simulink model "househeat"  (R2018b)
settings: Solver=ode15s  StartTime=0.0  StopTime=3600*24*55  FixedStep=1  RelTol=1e-3  AbsTol=1e-6
model workspace (MATLAB code in the model file):
  | % load initial conditions and physical properties from file
  | 
  | %sldemo_househeat_data
  | househeat_data_szakdoga
  | onlabmpc
  | 
  | 
  | addpath('subsystems')
  | 
  | %disp('adding models...')
  | load('subsystems/MPC-expert.mat')
  | %disp('done.')
values from neighbouring files (symbols this model uses):
  A_heater = 3.5    [househeat_data_szakdoga.m]
  c = 1005.4    [househeat_data_szakdoga.m]
  h_heater = 11    [househeat_data_szakdoga.m]
  M = (lenHouse*widHouse*htHouse+tan(pitRoof)*widHouse*lenHouse)*densAir    [househeat_data_szakdoga.m]
  Req = RWall*RWindow/(RWall + RWindow)    [househeat_data_szakdoga.m]
  T_s = 1800    [househeat_data_szakdoga.m]
  timeUnit_1week = 7*timeUnit_1day    (= 336)    [househeat_data_szakdoga.m]
  TinHeatK = 273    [househeat_data_szakdoga.m]
  TinIC = 0    [househeat_data_szakdoga.m]
undefined symbols (not defined in the file or in its folder): disturbance, f, FloorHeatFlowIn, RadiatorHeatFlow, RadiatorSurface, referenceSloped
libraries: fl_lib x39, nesl_utility x14, simulink x2, instrumentlib x2, mpclib x1, dspnetwork x1, powerlib_meascontrol x1
Description:
  | Thermal Model of a House
  | 
  | This demo illustrates how you can use Simulink(R) to create the thermal model of
  | a house. This system models the outdoor environment, the thermal
  | characteristics of the house, and the house heating system.
  | 
  | The sldemo_househeat_data.m file initializes data in the model workspace.
  | To make changes, you can edit the model workspace directly or edit the MATLAB(R) file
  | and re-load the model workspace.
  | 
  | To view the model workspace, select View > Model Explorer
  | from the Simulink editor.
  | 
  | Note: Time is given in units of hours
settings Model: SimulationMode=accelerator  PauseTimes=648000  NumberOfSteps=100  ExtModeTrigMode=oneshot  ExtModeArmWhenConnect=off  ExtModeAutoUpdateStatusClock=off  Creator=The MathWorks, Inc.  LastModifiedBy=Gyulai László
settings SolverCC: AutoScaleAbsTol=off
settings DataIOCC: ExternalInput=[]  InitialState=[]  SaveFormat=StructureWithTime  SaveOutput=off  SaveTime=off  SignalLoggingName=sldemo_househeat_output
settings OptimizationCC: BlockReduction=off  BooleanDataType=off  ExpressionDepthLimit=2147483647  InitFltsAndDblsToZero=on  EfficientMapNaN2IntZero=off  LifeSpan=inf  BufferReusableBoundary=off
settings DebuggingCC: SaveWithParameterizedLinksMsg=none  UnderspecifiedInitializationDetection=Classic  MergeDetectMultiDrivingBlocksExec=none  SignalResolutionControl=TryResolveAllWithWarning  MultiTaskDSMMsg=warning  MultiTaskCondExecSysMsg=none  IntegerOverflowMsg=none  FcnCallInpInsideContextMsg=warning  BusObjectLabelMismatch=none  StateNameClashWarn=warning  SFUnexpectedBacktrackingDiag=warning  SFNoUnconditionalDefaultTransitionDiag=warning  SFExecutionAtInitializationDiag=none  IntegerSaturationMsg=none
settings HardwareCC: ProdBitPerPointer=32  ProdBitPerSizeT=32  ProdBitPerPtrDiffT=32  ProdLargestAtomicFloat=None  ProdIntDivRoundTo=Undefined  ProdEndianess=Unspecified  ProdWordSize=32  ProdHWDeviceType=32-bit Generic  TargetBitPerPointer=64  TargetBitPerSizeT=64  TargetBitPerPtrDiffT=64  TargetLongLongMode=on  TargetIntDivRoundTo=Zero  TargetEndianess=LittleEndian  TargetWordSize=64  TargetHWDeviceType=MATLAB Host  ProdEqTarget=off
settings ModelReferenceCC: PropagateSignalLabelsOutOfModel=off
settings SFSimCC: SimUseLocalCustomCode=off
settings CodeAppCC: MaxIdLength=128
settings GRTTargetCC: TargetLangStandard=C89/C90 (ANSI)  CombineOutputUpdateFcns=off  GRTInterface=on
settings ConfigComp: CovMetricSettings=dw  CovHtmlReporting=on  CovSaveCumulativeToWorkspaceVar=on  CovSaveSingleToWorkspaceVar=on  CovExternalEMLEnable=off
settings SimscapeCC: SimscapeNormalizeSystem=off

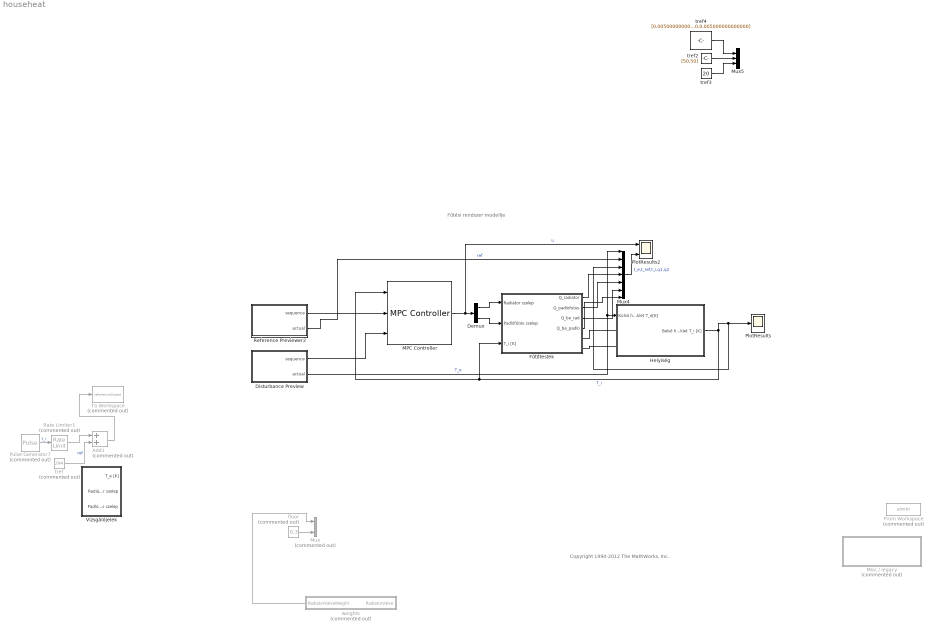
== system househeat ==
  note: Fűtési rendszer modellje
  note: Copyright 1990-2012 The MathWorks, Inc.
  Add1 : Sum  Commented=on
  Demux : Demux  Outputs=2
  Disturbance Preview : Subsystem  mask{signal=disturbance, ts=1800, steps=10}
      mask prompts: signal "Signal name"; ts "Sampling time"; steps "Number of previewing steps"
      mask init:
      | ts = evalin('base',get_param(gcbh,'ts'));
      | signal = evalin('base',get_param(gcbh,'signal'));
      | steps = evalin('base',get_param(gcbh,'steps'));
      | data = mpc_previewer_maskinit(signal,ts);
      mask Display:
      | fprintf('Future\nsample\nextractor');
      | port_label('output', 1, 'seq')
      | port_label('output', 2, '@t')
  From Workspace : FromWorkspace  Commented=on  VariableName=simin  SampleTime=0
  Fűtőtestek : Subsystem
  Helyiség : Subsystem
  MPC Controller : mpclib/MPC Controller  SCDEnableBlockLinearizationSpecification=on  mpcobj=C  x0=Cinitial  is_multiple=0  enable_value=0  return_u0=off  updateMPCinCallerWorkspace=on  md_inport=on  mv_inport=off  return_cost=off  return_mvseq=off  return_qpstatus=off  return_xseq=off  return_state=off  return_ovseq=off  state_inport=off  umin_inport=off  umax_inport=off  ymin_inport=off  ymax_inport=off  cc_inport=off  ywt_inport=off  uwt_inport=off  duwt_inport=off  rhoeps_inport=off  uref_inport=off  n_ts=1800  n_p=48  n_mv=2  n_md=1  n_ud=0  n_mo=1  n_uo=0  BlockDataType=double  SampleTimeInherited=off  switch_inport=off
  Misc / legacy : Subsystem  Commented=on
  Mux : Mux  Commented=on  Inputs=3
  Mux4 : Mux  Inputs=7
  Mux5 : Mux  Inputs=3
  PlotResults : Scope
  PlotResults2 : Scope  NumInputPorts=2
  Pulse Generator7 : DiscretePulseGenerator  Commented=on  Period=2*24  PulseWidth=30  PhaseDelay=14  SampleTime=1800
  Rate Limiter1 : RateLimiter  Commented=on  RisingSlewLimit=0.00007  FallingSlewLimit=-0.00025  SampleTimeMode=inherited
  Reference Previewer2 : Subsystem  mask{signal=referenceSloped, ts=1800, steps=1}
      mask prompts: signal "Signal name"; ts "Sampling time"; steps "Number of previewing steps"
      mask init:
      | ts = evalin('base',get_param(gcbh,'ts'));
      | signal = evalin('base',get_param(gcbh,'signal'));
      | steps = evalin('base',get_param(gcbh,'steps'));
      | data = mpc_previewer_maskinit(signal,ts);
      mask Display:
      | fprintf('Future\nsample\nextractor');
      | port_label('output', 1, 'seq')
      | port_label('output', 2, '@t')
  To Workspace : ToWorkspace  Commented=on  VariableName=referenceSloped  SaveFormat=Structure With Time  SampleTime=-1
      settings: Save2DSignal=2-D array (concatenate along first dimension)
  Vizsgálójelek : Subsystem
  floor : Constant  Commented=on  Value=0.3  SampleTime=300
  tref : Constant  Commented=on  Value=294  SampleTime=1800
  tref2 : Constant  Value=[50,50]  SampleTime=1800
  tref3 : Constant  Value=20  SampleTime=1800
  tref4 : Constant  Value=[0.005000000000000,0.005000000000000]  SampleTime=1800
  weights : Subsystem  Commented=on
  wires:
  weights/1(RadiatorValveWeight) -> Mux/1
  floor/1 -> Mux/3
  MPC Controller/1 -> PlotResults2/1, Demux/1  "u"
  tref3/1 -> Mux5/3
  tref2/1 -> Mux5/2
  Disturbance Preview/2(actual) -> Helyiség/1(Külső hőmérséklet T_e[K]), Mux4/1  "T_e"
  Helyiség/1(Belső hőmérséklet T_i [K]) -> MPC Controller/1, Fűtőtestek/3(T_i [K]), Mux4/3, PlotResults/1  "T_i"
  Mux4/1 -> PlotResults2/2  "t_e,t_ref,t_i,q1,q2"
  tref4/1 -> Mux5/1
  Fűtőtestek/1(Q_radiator) -> Mux4/4
  Demux/1 -> Fűtőtestek/1(Radiátor szelep)
  Demux/2 -> Fűtőtestek/2(Padlófűtés szelep)
  Fűtőtestek/2(Q_padlofutes) -> Mux4/5
  Pulse Generator7/1 -> Rate Limiter1/1  "t_i"
  Rate Limiter1/1 -> Add1/1
  Reference Previewer2/2(actual) -> Mux4/2  "ref"
  Add1/1 -> To Workspace/1
  Disturbance Preview/1(sequence) -> MPC Controller/3
  Fűtőtestek/3(Q_be_rad) -> Mux4/6
  Fűtőtestek/4(Q_be_padlo) -> Mux4/7
  tref/1 -> Add1/2  "ref"
  Reference Previewer2/1(sequence) -> MPC Controller/2
  connections:
  Helyiség/LConn1 -- Fűtőtestek/RConn1
  Helyiség/LConn2 -- Fűtőtestek/RConn2

== system househeat/Disturbance Preview ==
  MATLAB Function : MATLAB Function  TreatAsAtomicUnit=on
  Memory1 : Memory  InheritSampleTime=on  LinearizeAsDelay=on
  sequence : Outport
  actual : Outport  Port=2
  wires:
  MATLAB Function/2(first) -> actual/1
  MATLAB Function/3(next_t) -> Memory1/1
  Memory1/1 -> MATLAB Function/1(t)
  MATLAB Function/1(seq) -> sequence/1

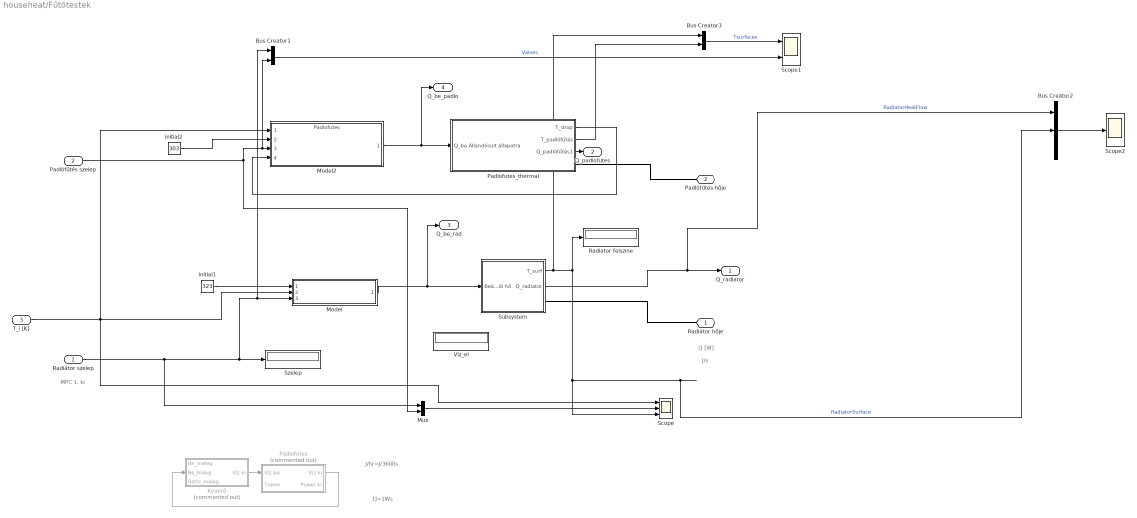
== system househeat/Fűtőtestek ==
  note: MPC 1. ki
  note: J/s
  note: 1J=1Ws
  note: J/hr=J/3600s
  note: Q [W]
  Radiátor szelep : Inport
  Padlófűtés szelep : Inport  Port=2
  T_i [K] : Inport  Port=3
  Bus Creator1 : BusCreator  Inputs=2
  Bus Creator2 : BusCreator  Inputs=RadiatorHeatFlow,RadiatorSurface,FloorHeatFlowIn
  Bus Creator3 : BusCreator  Inputs=2
  Keverő : Subsystem  Commented=on
  Model : ModelReference  ModelNameDialog=Radiator  SimulationMode=Normal  ModelReferenceVersion=1.31
  Model2 : ModelReference  ModelNameDialog=Padlofutes.slx  SimulationMode=Normal  ModelReferenceVersion=1.29
  Mux : Mux  Inputs=2
  Padlofutes : Subsystem  Commented=on
  Padlofutes_thermal : Subsystem
  Radiator felszine : Display
  Scope : Scope  NumInputPorts=3
  Scope1 : Scope  NumInputPorts=2
  Scope2 : Scope
  Subsystem : Subsystem
  Szelep : Display
  Víz_el : Display
  initial1 : Constant  Value=323
  initial2 : Constant  Value=303
  Radiátor hője : PMIOPort  Side=Right
  Padlófűtés hője : PMIOPort  Port=2  Side=Right
  Q_radiator : Outport
  Q_padlofutes : Outport  Port=2
  Q_be_rad : Outport  Port=3
  Q_be_padlo : Outport  Port=4
  wires:
  T_i [K]/1 -> Scope/1, Model/2, Model2/1
  initial1/1 -> Model/1
  Padlofutes/1(Víz ki) -> Keverő/2(Be_hideg)
  Keverő/1(Víz ki) -> Padlofutes/1(Víz be)
  Mux/1 -> Scope/2
  Padlófűtés szelep/1 -> Bus Creator1/2, Model2/3, Mux/2
  Model2/1 -> Q_be_padlo/1, Padlofutes_thermal/1(Q_be Állandósult állapotra)
  Padlofutes_thermal/1(T_drop) -> Model2/4
  initial2/1 -> Model2/2
  ? -> Víz_el/1
  Bus Creator1/1 -> Scope1/2  "Valves"
  Bus Creator3/1 -> Scope1/1  "Tsurfaces"
  Radiátor szelep/1 -> Mux/1, Szelep/1, Bus Creator1/1, Model/3
  Padlofutes_thermal/2(T_padlófűtés) -> Bus Creator3/2
  Bus Creator2/1 -> Scope2/1
  Subsystem/1(T_surf) -> Bus Creator3/1, Bus Creator2/2, Scope/3, Radiator felszine/1  "RadiatorSurface"
  ? -> Bus Creator2/3  "FloorHeatFlowIn"
  Subsystem/2(Q_radiator) -> Q_radiator/1, Bus Creator2/1  "RadiatorHeatFlow"
  Padlofutes_thermal/3(Q_padlófűtés1) -> Q_padlofutes/1
  Model/1 -> Q_be_rad/1, Subsystem/1(Beáramló hő)
  connections:
  Radiátor hője/RConn1 -- Subsystem/RConn1
  Padlofutes_thermal/RConn1 -- Padlófűtés hője/RConn1

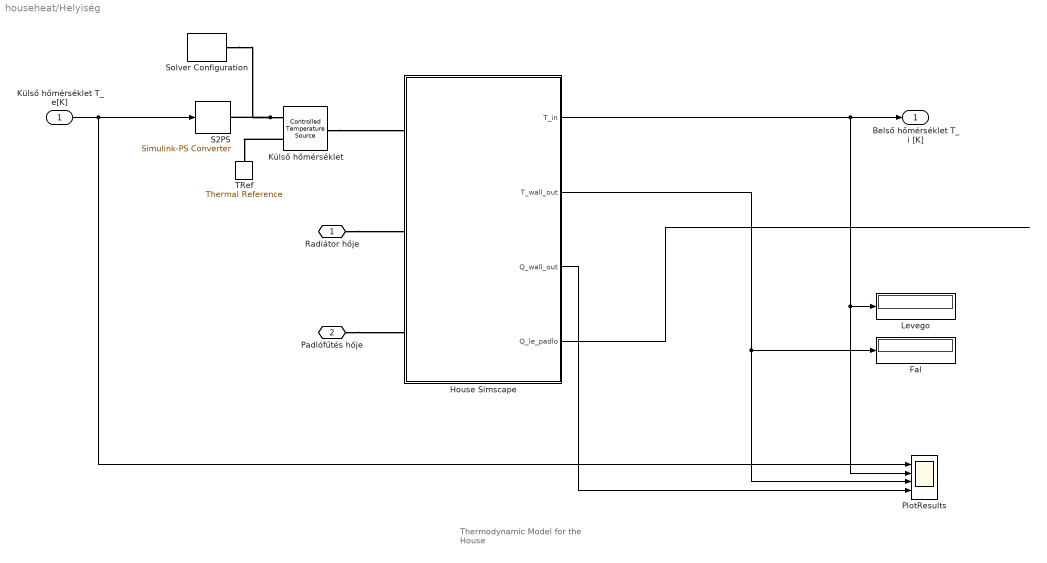
== system househeat/Helyiség ==
  note: Thermodynamic Model
      | for the House
  Külső hőmérséklet T_e[K] : Inport
  Fal : Display
  House Simscape : Subsystem
  Külső hőmérséklet : fl_lib/Thermal/Thermal Sources/Controlled Temperature Source
      settings: SourceProductName=Simscape
  Levego : Display
  PlotResults : Scope  NumInputPorts=4
  S2PS : nesl_utility/Simulink-PS Converter  PhysicalDomain=network_engine_domain  SubClassName=ps_input  LeftPortType=input  RightPortType=output  PseudoPeriodic=off  Frequencies=[]  NoiseDistribution=none  NoiseParameters=[]  Unit=1  AffineConversion=off  FilteringAndDerivatives=zero  SimscapeFilterOrder=1  InputFilterTimeConstant=.001  UdotUserProvided=0
  Solver Configuration : nesl_utility/Solver Configuration  PhysicalDomain=network_engine_domain  SubClassName=solver  LeftPortType=input  RightPortType=generic  Tones=[]  Harmonics=[]  SimulateNoise=off  Profile=off  UseLocalSampling=off  EnableSwitchedLinearOptims=on  FrequencyDomain=off  UseCCode=off  RelTol=0.001  AbsTol=1e-06  MinStep=1e-09  ToWorkspace=off  RevertToSquareIcSolve=off  NumHomotopyIterations=100  PhasorMode=off  PhasorModeNumHarmonics=1  DoDC=off  ResidualTolerance=1e-9  UseLocalSolver=off  LocalSolverChoice=NE_BACKWARD_EULER_ADVANCER  LocalSolverSampleTime=.001  DoFixedCost=off  MaxNonlinIter=3  MaxModeIter=2  LinearAlgebra=Sparse  EquationFormulation=NE_TIME_EF  DelaysMemoryBudget=1024  AutomaticFiltering=on  FilteringTimeConstant=0.001  PartitionStorageMethod=AS_NEEDED  PartitionMemoryBudget=1024
  TRef : fl_lib/Thermal/Thermal Elements/Thermal Reference
  Radiátor hője : PMIOPort  Side=Left
  Padlófűtés hője : PMIOPort  Port=2  Side=Left
  Belső hőmérséklet T_i [K] : Outport  InitialOutput=0
  wires:
  House Simscape/3(Q_wall_out) -> PlotResults/4
  House Simscape/1(T_in) -> PlotResults/2, Levego/1, Belső hőmérséklet T_i [K]/1
  House Simscape/2(T_wall_out) -> Fal/1, PlotResults/3
  Külső hőmérséklet T_e[K]/1 -> S2PS/1, PlotResults/1
  House Simscape/4(Q_le_padlo) -> ?
  connections:
  Radiátor hője/RConn1 -- House Simscape/LConn2
  Külső hőmérséklet/RConn1 -- Solver Configuration/RConn1 -- S2PS/RConn1
  Külső hőmérséklet/LConn1 -- House Simscape/LConn1
  Külső hőmérséklet/RConn2 -- TRef/LConn1
  Padlófűtés hője/RConn1 -- House Simscape/LConn3

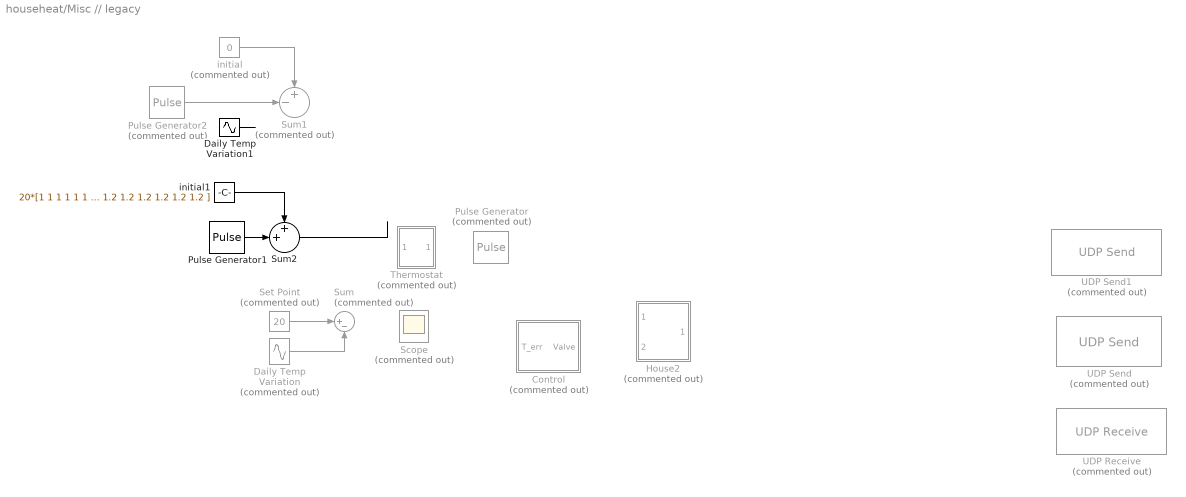
== system househeat/Misc // legacy ==
  Control : Subsystem  Commented=on
  Daily Temp Variation : Sin  Commented=on  Amplitude=5  Frequency=3.14*2/3600/24  Phase=3.14/2  SampleTime=0
  Daily Temp Variation1 : Sin  Amplitude=5  Frequency=3.14*2/3600/24  Phase=3.14/2  SampleTime=300
  House2 : Subsystem  Commented=on
      mask Display: image(fullfile(matlabroot,'toolbox','simulink','simdemos','simgeneral','images','HouseHeatHousePix.svg'))
  Pulse Generator : DiscretePulseGenerator  Commented=on  PulseType=Time based  Period=3600*24*4  PulseWidth=50
  Pulse Generator1 : DiscretePulseGenerator  Amplitude=0  Period=12*24  PulseWidth=12  SampleTime=300
  Pulse Generator2 : DiscretePulseGenerator  Commented=on  Amplitude=0  Period=12*24  PulseWidth=12*4  SampleTime=300
  Scope : Scope  Commented=on
  Set Point : Constant  Commented=on  Value=20
  Sum : Sum  Commented=on  Inputs=+-|  SaturateOnIntegerOverflow=on  InputSameDT=on  OutDataTypeStr=Inherit: Same as first input
  Sum1 : Sum  Commented=on  Inputs=+-|  SaturateOnIntegerOverflow=on  InputSameDT=on  OutDataTypeStr=Inherit: Same as first input
  Sum2 : Sum  Inputs=++|  SaturateOnIntegerOverflow=on  InputSameDT=on  OutDataTypeStr=Inherit: Same as first input
  Thermostat : Subsystem  Commented=on
      mask Display: image(fullfile(matlabroot,'toolbox','simulink','simdemos','simgeneral','images','HouseHeatThermostatPix.svg'))
  UDP Receive : instrumentlib/UDP Receive  Commented=on  Host=localhost  Port=9090  LocalPort=-1  EnablePortSharing=off  GetLatestData=off  DataSize=[1 1]  DataType=uint8  ASCIIFormatting=%f,  Terminator=LF  ByteOrder=BigEndian  EnableBlockingMode=on  Timeout=10  SampleTime=0.01  LocalAddress=0.0.0.0
      settings: SourceProductName=Instrument Control Toolbox
  UDP Send : dspnetwork/UDP Send  Commented=on  remoteURL='127.0.0.1'  remotePort=25000  localURL='0.0.0.0'  localPortSource=Automatically determine  localPort=-1  sampletime=-1  blockPlatform=[]  separateLengthPort=0
      settings: SourceProductName=DSP System Toolbox  SourceProductBaseCode=DS
  UDP Send1 : instrumentlib/UDP Send  Commented=on  Port=9090  LocalPort=-1  EnablePortSharing=off  ByteOrder=BigEndian  OutputDatagramPacketSize=512  EnableBlockingMode=on  LocalAddress=0.0.0.0
      settings: SourceProductName=Instrument Control Toolbox
  initial : Constant  Commented=on  Value=0  SampleTime=300
  initial1 : Constant  Value=20*[1 1 1 1 1 1 1 1 1 1 1 1 1 1 1 1 1 1 1 1 1 1 1 1 1.2 1.2 1.2 1.2 1.2 1.2 1.2 1.2 1.2 1.2 1.2 1.2 1.2 1.2 1.2 1.2 1.2 1.2 1.2 1.2 1.2 1.2 1.2 1.2 ]  SampleTime=300
  wires:
  Set Point/1 -> Sum/1
  Daily Temp Variation/1 -> Sum/2
  Pulse Generator1/1 -> Sum2/2
  Pulse Generator2/1 -> Sum1/2
  initial1/1 -> Sum2/1
  Daily Temp Variation1/1 -> ?
  initial/1 -> Sum1/1
  Sum2/1 -> ?

== system househeat/Reference Previewer2 ==
  MATLAB Function : MATLAB Function  TreatAsAtomicUnit=on
  Memory1 : Memory  InheritSampleTime=on  LinearizeAsDelay=on
  sequence : Outport
  actual : Outport  Port=2
  wires:
  MATLAB Function/2(first) -> actual/1
  MATLAB Function/3(next_t) -> Memory1/1
  Memory1/1 -> MATLAB Function/1(t)
  MATLAB Function/1(seq) -> sequence/1

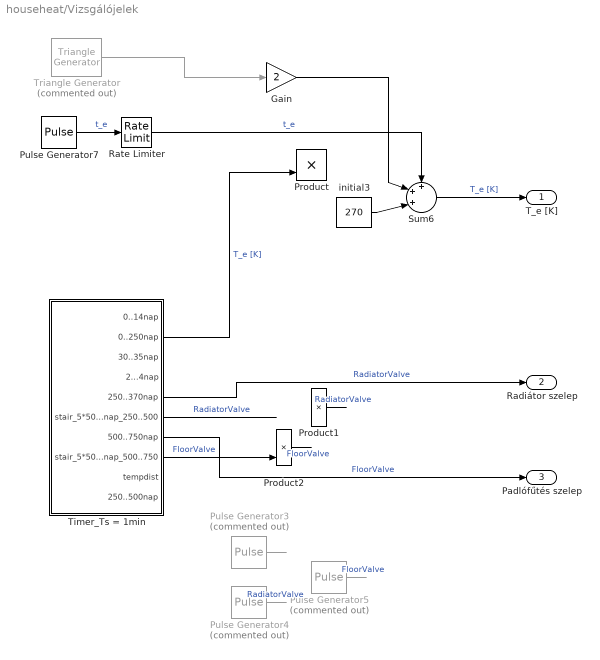
== system househeat/Vizsgálójelek ==
  Gain : Gain  Gain=2
  Product : Product
  Product1 : Product
  Product2 : Product
  Pulse Generator3 : DiscretePulseGenerator  Commented=on  PulseType=Time based  Period=3600*24*30*3  PulseWidth=45  PhaseDelay=3600*24*20
  Pulse Generator4 : DiscretePulseGenerator  Commented=on  PulseType=Time based  Amplitude=0.5  Period=3600*24*30*3  PulseWidth=50
  Pulse Generator5 : DiscretePulseGenerator  Commented=on  PulseType=Time based  Period=3600*24*30*3  PulseWidth=40
  Pulse Generator7 : DiscretePulseGenerator  Amplitude=10  Period=2*24  PulseWidth=16  PhaseDelay=20  SampleTime=1800
  Rate Limiter : RateLimiter  RisingSlewLimit=0.0005  FallingSlewLimit=-0.0005  SampleTimeMode=inherited
  Sum6 : Sum  Inputs=+++|  SaturateOnIntegerOverflow=on  InputSameDT=on  OutDataTypeStr=Inherit: Same as first input
  Timer_Ts = 1min : Subsystem
  Triangle Generator : powerlib_meascontrol/Pulse & Signal Generators/Triangle Generator  Commented=on  Freq=1/(3600*24*30)  Phase=210  Ts=1800
      settings: SourceProductName=Simscape Electrical
  initial3 : Constant  Value=270  SampleTime=1800
  T_e [K] : Outport
  Radiátor szelep : Outport  Port=2
  Padlófűtés szelep : Outport  Port=3
  wires:
  Product1/1 -> ?  "RadiatorValve"
  Timer_Ts = 1min/2(0..250nap) -> Product/2  "T_e [K]"
  initial3/1 -> Sum6/3
  Rate Limiter/1 -> Sum6/1  "t_e"
  Timer_Ts = 1min/6(stair_5*50nap_250..500) -> ?  "RadiatorValve"
  ? -> Product2/1
  Triangle Generator/1 -> Gain/1
  ? -> Product1/1
  Timer_Ts = 1min/8(stair_5*50nap_500..750) -> Product2/2  "FloorValve"
  Sum6/1 -> T_e [K]/1  "T_e [K]"
  Timer_Ts = 1min/5(250..370nap) -> Radiátor szelep/1  "RadiatorValve"
  Timer_Ts = 1min/7(500..750nap) -> Padlófűtés szelep/1  "FloorValve"
  Pulse Generator5/1 -> ?  "FloorValve"
  ? -> Product1/2
  Pulse Generator3/1 -> ?
  Product2/1 -> ?  "FloorValve"
  Pulse Generator4/1 -> ?  "RadiatorValve"
  Gain/1 -> Sum6/2
  Pulse Generator7/1 -> Rate Limiter/1  "t_e"

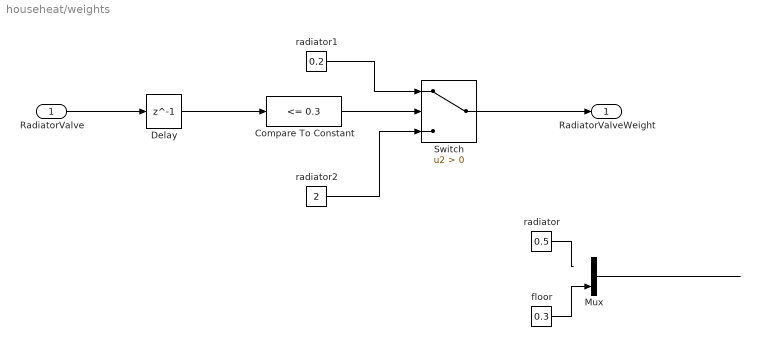
== system househeat/weights ==
  RadiatorValve : Inport
  Compare To Constant : simulink/Logic and Bit Operations/Compare To Constant  relop=<=  const=0.3  OutDataTypeStr=boolean
  Delay : Delay  DelayLength=1  InitialCondition=0
  Mux : Mux  Inputs=2
  Switch : Switch  Criteria=u2 > Threshold
  floor : Constant  Value=0.3
  radiator : Constant  Value=0.5
  radiator1 : Constant  Value=0.2  SampleTime=300
  radiator2 : Constant  Value=2  SampleTime=300
  RadiatorValveWeight : Outport
  wires:
  Mux/1 -> ?
  radiator/1 -> ?
  floor/1 -> Mux/2
  Compare To Constant/1 -> Switch/2
  radiator1/1 -> Switch/1
  radiator2/1 -> Switch/3
  Switch/1 -> RadiatorValveWeight/1
  RadiatorValve/1 -> Delay/1
  Delay/1 -> Compare To Constant/1

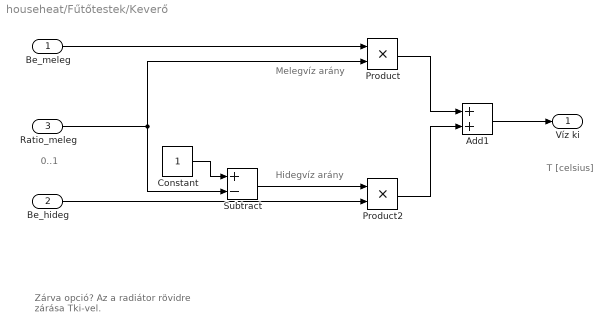
== system househeat/Fűtőtestek/Keverő ==
  note: T [celsius]
  note: Hidegvíz arány
  note: Zárva opció?
      | Az a radiátor rövidre zárása Tki-vel.
  note: 0..1
  note: Melegvíz arány
  Be_meleg : Inport
  Be_hideg : Inport  Port=2
  Ratio_meleg : Inport  Port=3
  Add1 : Sum
  Constant : Constant
  Product : Product
  Product2 : Product
  Subtract : Sum  Inputs=+-
  Víz ki : Outport
  wires:
  Be_meleg/1 -> Product/1
  Ratio_meleg/1 -> Subtract/2, Product/2
  Constant/1 -> Subtract/1
  Be_hideg/1 -> Product2/2
  Subtract/1 -> Product2/1
  Product/1 -> Add1/1
  Product2/1 -> Add1/2
  Add1/1 -> Víz ki/1

== system househeat/Fűtőtestek/Padlofutes ==
  note: Ide johet a radiátor karakterisztika a felszín hőmérsékletéhez
  note: Feluleti homerseklet ----- képlet van a HERZ II-ban!
  Víz be : Inport
  Troom : Inport  Port=2
  Radiátor : Gain  Gain=A_heater*h_heater
  Víz ki : Outport
  Power ki : Outport  Port=2
  wires:
  Víz be/1 -> Víz ki/1

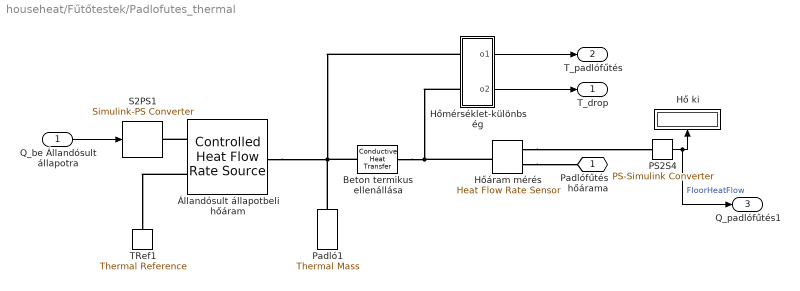
== system househeat/Fűtőtestek/Padlofutes_thermal ==
  Q_be Állandósult állapotra : Inport
  Beton termikus ellenállása : fl_lib/Thermal/Thermal Elements/Conductive Heat Transfer  area=15 m^2  thickness=0.05 m  th_cond=1.2 W/(m*K)  T_specify=off  T_priority=None  T=0 K  T_nominal_specify=off  T_nominal_unit=K  T_nominal_value=1  Q_specify=off  Q_priority=None  Q=0 J/s  Q_nominal_specify=off  Q_nominal_unit=W  Q_nominal_value=1
      settings: SourceProductName=Simscape
  Hő ki : Display
  Hőmérséklet-különbség : Subsystem
  Hőáram mérés : fl_lib/Thermal/Thermal Sensors/Heat Flow Rate Sensor
      settings: SourceProductName=Simscape  SourceProductBaseCode=SS
  PS2S4 : nesl_utility/PS-Simulink Converter  PhysicalDomain=network_engine_domain  SubClassName=ps_output  LeftPortType=input  RightPortType=output  PseudoPeriodic=off  Frequencies=[]  Unit=J/s  AffineConversion=on
  Padló1 : fl_lib/Thermal/Thermal Elements/Thermal Mass  mass=1000 kg  sp_heat=840 J/kg/K  T_specify=on  T_priority=High  T=TinIC degC  T_nominal_specify=off  T_nominal_unit=K  T_nominal_value=1  Q_specify=off  Q_priority=None  Q=0 J/s  Q_nominal_specify=off  Q_nominal_unit=W  Q_nominal_value=1
      settings: LogSimulationData=on
  S2PS1 : nesl_utility/Simulink-PS Converter  PhysicalDomain=network_engine_domain  SubClassName=ps_input  LeftPortType=input  RightPortType=output  PseudoPeriodic=off  Frequencies=[]  NoiseDistribution=none  NoiseParameters=[]  Unit=1  AffineConversion=off  FilteringAndDerivatives=zero  SimscapeFilterOrder=1  InputFilterTimeConstant=.001  UdotUserProvided=0
  TRef1 : fl_lib/Thermal/Thermal Elements/Thermal Reference
  Állandósult állapotbeli hőáram : fl_lib/Thermal/Thermal Sources/Controlled Heat Flow Rate Source
      settings: SourceProductName=Simscape
  Padlófűtés hőárama : PMIOPort  Side=Right
  T_drop : Outport
  T_padlófűtés : Outport  Port=2
  Q_padlófűtés1 : Outport  Port=3
  wires:
  Q_be Állandósult állapotra/1 -> S2PS1/1
  PS2S4/1 -> Q_padlófűtés1/1, Hő ki/1  "FloorHeatFlow"
  Hőmérséklet-különbség/1(o1) -> T_padlófűtés/1
  Hőmérséklet-különbség/2(o2) -> T_drop/1
  connections:
  Beton termikus ellenállása/RConn1 -- Hőmérséklet-különbség/LConn2 -- Hőáram mérés/LConn1
  Beton termikus ellenállása/LConn1 -- Állandósult állapotbeli hőáram/LConn1 -- Hőmérséklet-különbség/LConn1 -- Padló1/LConn1
  Állandósult állapotbeli hőáram/RConn1 -- S2PS1/RConn1
  Állandósult állapotbeli hőáram/RConn2 -- TRef1/LConn1
  Hőáram mérés/RConn2 -- Padlófűtés hőárama/RConn1
  Hőáram mérés/RConn1 -- PS2S4/LConn1

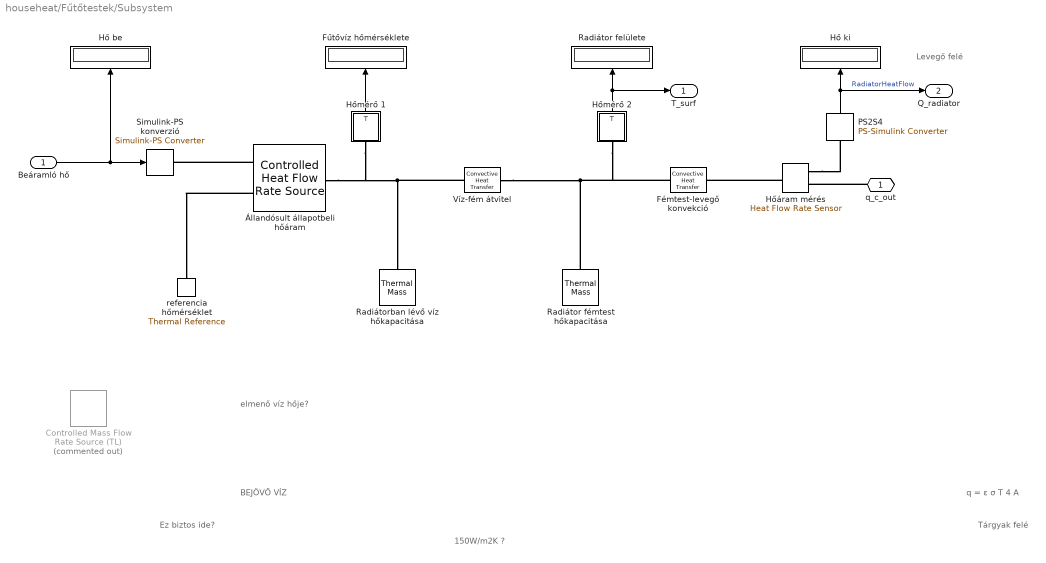
== system househeat/Fűtőtestek/Subsystem ==
  note: elmenő víz hője?
  note: BEJÖVŐ VÍZ
  note: q = ε σ T 4 A
  note: 150W/m2K ?
  note: Tárgyak felé
  note: Levegő felé
  note: Ez biztos ide?
  Beáramló hő : Inport
  Controlled Mass Flow Rate Source (TL) : fl_lib/Thermal Liquid/Sources/Controlled Mass Flow Rate Source (TL)  Commented=on  area=0.01 m^2  length=0.1 m  mdot_A_specify=off  mdot_A_priority=None  mdot_A=1 kg/s  mdot_A_nominal_specify=off  mdot_A_nominal_unit=kg/s  mdot_A_nominal_value=1
      settings: SourceProductName=Simscape  SourceProductBaseCode=SS
  Fémtest-levegő konvekció : fl_lib/Thermal/Thermal Elements/Convective Heat Transfer  area=area_radiator m^2  heat_tr_coeff=h_c_radi W/(m^2 * K)  T_specify=off  T_priority=None  T=0 K  T_nominal_specify=off  T_nominal_unit=K  T_nominal_value=1  Q_specify=off  Q_priority=None  Q=0 J/s  Q_nominal_specify=off  Q_nominal_unit=W  Q_nominal_value=1
  Fűtővíz hőmérséklete : Display
  Hő be : Display
  Hő ki : Display
  Hőmérő 1 : Subsystem
  Hőmérő 2 : Subsystem
  Hőáram mérés : fl_lib/Thermal/Thermal Sensors/Heat Flow Rate Sensor
      settings: SourceProductName=Simscape  SourceProductBaseCode=SS
  PS2S4 : nesl_utility/PS-Simulink Converter  PhysicalDomain=network_engine_domain  SubClassName=ps_output  LeftPortType=input  RightPortType=output  PseudoPeriodic=off  Frequencies=[]  Unit=J/s  AffineConversion=on
  Radiátor felülete : Display
  Radiátor fémtest hőkapacitása : fl_lib/Thermal/Thermal Elements/Thermal Mass  mass=m_r kg  sp_heat=c_metal J/kg/K  T_specify=on  T_priority=High  T=TinHeatK K  T_nominal_specify=off  T_nominal_unit=K  T_nominal_value=1  Q_specify=off  Q_priority=None  Q=0 J/s  Q_nominal_specify=off  Q_nominal_unit=W  Q_nominal_value=1
  Radiátorban lévő víz hőkapacitása : fl_lib/Thermal/Thermal Elements/Thermal Mass  mass=m_w_r kg  sp_heat=c_w J/kg/K  T_specify=on  T_priority=High  T=TinHeatK K  T_nominal_specify=off  T_nominal_unit=K  T_nominal_value=1  Q_specify=off  Q_priority=None  Q=0 J/s  Q_nominal_specify=off  Q_nominal_unit=W  Q_nominal_value=1
  Simulink-PS konverzió : nesl_utility/Simulink-PS Converter  PhysicalDomain=network_engine_domain  SubClassName=ps_input  LeftPortType=input  RightPortType=output  PseudoPeriodic=off  Frequencies=[]  NoiseDistribution=none  NoiseParameters=[]  Unit=1  AffineConversion=off  FilteringAndDerivatives=zero  SimscapeFilterOrder=1  InputFilterTimeConstant=0.001  UdotUserProvided=1
  Víz-fém átvitel : fl_lib/Thermal/Thermal Elements/Convective Heat Transfer  area=area_radiator m^2  heat_tr_coeff=h_w_radi W/(m^2 * K)  T_specify=off  T_priority=None  T=0 K  T_nominal_specify=off  T_nominal_unit=K  T_nominal_value=1  Q_specify=off  Q_priority=None  Q=0 J/s  Q_nominal_specify=off  Q_nominal_unit=W  Q_nominal_value=1
  referencia hőmérséklet : fl_lib/Thermal/Thermal Elements/Thermal Reference
  Állandósult állapotbeli hőáram : fl_lib/Thermal/Thermal Sources/Controlled Heat Flow Rate Source
      settings: SourceProductName=Simscape
  q_c_out : PMIOPort  Side=Right
  T_surf : Outport
  Q_radiator : Outport  Port=2
  wires:
  Beáramló hő/1 -> Simulink-PS konverzió/1, Hő be/1
  Hőmérő 2/1(T) -> Radiátor felülete/1, T_surf/1
  Hőmérő 1/1(T) -> Fűtővíz hőmérséklete/1
  PS2S4/1 -> Hő ki/1, Q_radiator/1  "RadiatorHeatFlow"
  connections:
  Állandósult állapotbeli hőáram/RConn1 -- Simulink-PS konverzió/RConn1
  Radiátor fémtest hőkapacitása/LConn1 -- Fémtest-levegő konvekció/LConn1 -- Hőmérő 2/LConn1 -- Víz-fém átvitel/RConn1
  Víz-fém átvitel/LConn1 -- Állandósult állapotbeli hőáram/LConn1 -- Hőmérő 1/LConn1 -- Radiátorban lévő víz hőkapacitása/LConn1
  Állandósult állapotbeli hőáram/RConn2 -- referencia hőmérséklet/LConn1
  Hőáram mérés/RConn1 -- PS2S4/LConn1
  q_c_out/RConn1 -- Hőáram mérés/RConn2
  Hőáram mérés/LConn1 -- Fémtest-levegő konvekció/RConn1

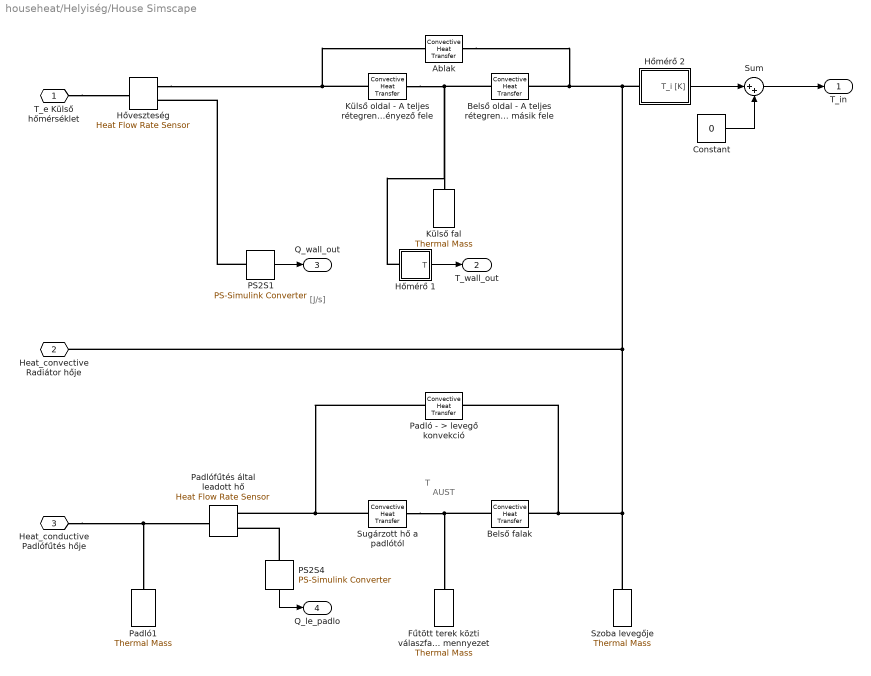
== system househeat/Helyiség/House Simscape ==
  note: T
  note: AUST
  note: [J/s]
  Ablak : fl_lib/Thermal/Thermal Elements/Convective Heat Transfer  area=4 m^2  heat_tr_coeff=4 W/(m^2 * K)  T_specify=off  T_priority=None  T=0 K  T_nominal_specify=off  T_nominal_unit=K  T_nominal_value=1  Q_specify=off  Q_priority=None  Q=0 J/s  Q_nominal_specify=off  Q_nominal_unit=W  Q_nominal_value=1
  Belső falak : fl_lib/Thermal/Thermal Elements/Convective Heat Transfer  area=65 m^2  heat_tr_coeff=7 W/(m^2 * K)  T_specify=off  T_priority=None  T=0 K  T_nominal_specify=off  T_nominal_unit=K  T_nominal_value=1  Q_specify=off  Q_priority=None  Q=0 J/s  Q_nominal_specify=off  Q_nominal_unit=W  Q_nominal_value=1
  Belső oldal - A teljes rétegrendi hőátbocsátási tényező másik fele : fl_lib/Thermal/Thermal Elements/Convective Heat Transfer  area=4.5 m^2  heat_tr_coeff=8 W/(m^2 * K)  T_specify=off  T_priority=None  T=0 K  T_nominal_specify=off  T_nominal_unit=K  T_nominal_value=1  Q_specify=off  Q_priority=None  Q=0 J/s  Q_nominal_specify=off  Q_nominal_unit=W  Q_nominal_value=1
  Constant : Constant  Value=0
  "Fűtött terek közti válaszfalak, mennyezet" : fl_lib/Thermal/Thermal Elements/Thermal Mass  mass=6000 kg  sp_heat=840 J/kg/K  T_specify=on  T_priority=High  T=TinIC degC  T_nominal_specify=off  T_nominal_unit=K  T_nominal_value=1  Q_specify=off  Q_priority=None  Q=0 J/s  Q_nominal_specify=off  Q_nominal_unit=W  Q_nominal_value=1
      settings: LogSimulationData=on
  Hőmérő 1 : Subsystem
  Hőmérő 2 : Subsystem
  Hőveszteség : fl_lib/Thermal/Thermal Sensors/Heat Flow Rate Sensor
      settings: SourceProductName=Simscape  SourceProductBaseCode=SS
  Külső fal : fl_lib/Thermal/Thermal Elements/Thermal Mass  mass=1200 kg  sp_heat=840 J/kg/K  T_specify=on  T_priority=High  T=TinIC degC  T_nominal_specify=off  T_nominal_unit=K  T_nominal_value=1  Q_specify=off  Q_priority=None  Q=0 J/s  Q_nominal_specify=off  Q_nominal_unit=W  Q_nominal_value=1
      settings: LogSimulationData=on
  Külső oldal - A teljes rétegrendi hőátbocsátási tényező fele : fl_lib/Thermal/Thermal Elements/Convective Heat Transfer  area=4.5 m^2  heat_tr_coeff=0.6 W/(m^2 * K)  T_specify=off  T_priority=None  T=0 K  T_nominal_specify=off  T_nominal_unit=K  T_nominal_value=1  Q_specify=off  Q_priority=None  Q=0 J/s  Q_nominal_specify=off  Q_nominal_unit=W  Q_nominal_value=1
  PS2S1 : nesl_utility/PS-Simulink Converter  PhysicalDomain=network_engine_domain  SubClassName=ps_output  LeftPortType=input  RightPortType=output  PseudoPeriodic=off  Frequencies=[]  Unit=J/s  AffineConversion=on
  PS2S4 : nesl_utility/PS-Simulink Converter  PhysicalDomain=network_engine_domain  SubClassName=ps_output  LeftPortType=input  RightPortType=output  PseudoPeriodic=off  Frequencies=[]  Unit=J/s  AffineConversion=on
  Padló - > levegő konvekció : fl_lib/Thermal/Thermal Elements/Convective Heat Transfer  area=16 m^2  heat_tr_coeff=4 W/(m^2 * K)  T_specify=off  T_priority=None  T=0 K  T_nominal_specify=off  T_nominal_unit=K  T_nominal_value=1  Q_specify=off  Q_priority=None  Q=0 J/s  Q_nominal_specify=off  Q_nominal_unit=W  Q_nominal_value=1
  Padló1 : fl_lib/Thermal/Thermal Elements/Thermal Mass  mass=1000 kg  sp_heat=840 J/kg/K  T_specify=on  T_priority=High  T=TinIC degC  T_nominal_specify=off  T_nominal_unit=K  T_nominal_value=1  Q_specify=off  Q_priority=None  Q=0 J/s  Q_nominal_specify=off  Q_nominal_unit=W  Q_nominal_value=1
      settings: LogSimulationData=on
  Padlófűtés által leadott hő : fl_lib/Thermal/Thermal Sensors/Heat Flow Rate Sensor
      settings: SourceProductName=Simscape  SourceProductBaseCode=SS
  Sugárzott hő a padlótól : fl_lib/Thermal/Thermal Elements/Convective Heat Transfer  area=16 m^2  heat_tr_coeff=5.4 W/(m^2 * K)  T_specify=off  T_priority=None  T=0 K  T_nominal_specify=off  T_nominal_unit=K  T_nominal_value=1  Q_specify=off  Q_priority=None  Q=0 J/s  Q_nominal_specify=off  Q_nominal_unit=W  Q_nominal_value=1
  Sum : Sum  Inputs=|++
  Szoba levegője : fl_lib/Thermal/Thermal Elements/Thermal Mass  mass=M_air kg  sp_heat=c_air J/kg/K  T_specify=on  T_priority=High  T=TinIC degC  T_nominal_specify=off  T_nominal_unit=K  T_nominal_value=1  Q_specify=off  Q_priority=None  Q=0 J/s  Q_nominal_specify=off  Q_nominal_unit=W  Q_nominal_value=1
  T_e Külső hőmérséklet : PMIOPort  Side=Left
  Heat_convective Radiátor hője : PMIOPort  Port=2  Side=Left
  Heat_conductive Padlófűtés hője : PMIOPort  Port=3  Side=Left
  T_in : Outport
  T_wall_out : Outport  Port=2
  Q_wall_out : Outport  Port=3
  Q_le_padlo : Outport  Port=4
  wires:
  PS2S1/1 -> Q_wall_out/1
  PS2S4/1 -> Q_le_padlo/1
  Hőmérő 1/1(T) -> T_wall_out/1
  Hőmérő 2/1(T_i [K]) -> Sum/1
  Sum/1 -> T_in/1
  Constant/1 -> Sum/2
  connections:
  Külső oldal - A teljes rétegrendi hőátbocsátási tényező fele/RConn1 -- Belső oldal - A teljes rétegrendi hőátbocsátási tényező másik fele/LConn1 -- Hőmérő 1/LConn1 -- Külső fal/LConn1
  Külső oldal - A teljes rétegrendi hőátbocsátási tényező fele/LConn1 -- Ablak/LConn1 -- Hőveszteség/RConn2
  Padló - > levegő konvekció/LConn1 -- Sugárzott hő a padlótól/LConn1 -- Padlófűtés által leadott hő/RConn2
  Belső falak/RConn1 -- Sugárzott hő a padlótól/RConn1 -- "Fűtött terek közti válaszfalak, mennyezet"/LConn1
  PS2S1/LConn1 -- Hőveszteség/RConn1
  Szoba levegője/LConn1 -- Belső falak/LConn1 -- Padló - > levegő konvekció/RConn1 -- Hőmérő 2/LConn1 -- Ablak/RConn1 -- Belső oldal - A teljes rétegrendi hőátbocsátási tényező másik fele/RConn1 -- Heat_convective Radiátor hője/RConn1
  PS2S4/LConn1 -- Padlófűtés által leadott hő/RConn1
  Heat_conductive Padlófűtés hője/RConn1 -- Padlófűtés által leadott hő/LConn1 -- Padló1/LConn1
  T_e Külső hőmérséklet/RConn1 -- Hőveszteség/LConn1

== system househeat/Misc // legacy/Control ==
  note: valve opening rate
  T_err : Inport
  PID Controller : simulink/Continuous/PID Controller  Controller=PI  Form=Parallel  TimeDomain=Continuous-time  SampleTime=-1  IntegratorMethod=Forward Euler  FilterMethod=Forward Euler  ControllerParametersSource=internal  P=0.09  I=9.95e-07  D=0  UseFilter=on  N=100  TunerSelectOption=Transfer Function Based (PID Tuner App)  InitialConditionSource=internal  InitialConditionForIntegrator=0  InitialConditionForFilter=0  DifferentiatorICPrevScaledInput=0  ExternalReset=none  TrackingMode=off  Kt=1  LimitOutput=on  UpperSaturationLimit=1  LowerSaturationLimit=0  LinearizeAsGain=on  AntiWindupMode=none  Kb=1  POutMin=[]  POutMax=[]  IOutMin=[]  IOutMax=[]  DOutMin=[]  DOutMax=[]  NOutMin=[]  NOutMax=[]  SumOutMin=[]  SumOutMax=[]  SaturationOutMin=[]  SaturationOutMax=[]  PParamMin=[]  PParamMax=[]  IParamMin=[]  IParamMax=[]  DParamMin=[]  DParamMax=[]  NParamMin=[]  NParamMax=[]  KbParamMin=[]  KbParamMax=[]  KtParamMin=[]  KtParamMax=[]  KbOutMin=[]  KbOutMax=[]  KtOutMin=[]  KtOutMax=[]  IntegratorOutMin=[]  IntegratorOutMax=[]  FilterOutMin=[]  FilterOutMax=[]  SumI1OutMin=[]  SumI1OutMax=[]  SumI2OutMin=[]  SumI2OutMax=[]  SumI3OutMin=[]  SumI3OutMax=[]  SumI4OutMin=[]  SumI4OutMax=[]  SumDOutMin=[]  SumDOutMax=[]  DifferentiatorOutMin=[]  DifferentiatorOutMax=[]  FilterDiffOutCoefMin=[]  FilterDiffOutCoefMax=[]  ReciprocalOutMin=[]  ReciprocalOutMax=[]  SumDenOutMin=[]  SumDenOutMax=[]  SumNumOutMin=[]  SumNumOutMax=[]  DivideOutMin=[]  DivideOutMax=[]  IntegratorContinuousStateAttributes=''  IntegratorStateMustResolveToSignalObject=off  IntegratorRTWStateStorageClass=Auto  FilterContinuousStateAttributes=''  FilterStateMustResolveToSignalObject=off  FilterRTWStateStorageClass=Auto  ParallelPVariant=InternalParameters  IdealPVariant=Disabled  IVariant=InternalParameters  DVariant=Disabled  IntegratorVariant=Continuous  SatVariant=Enabled  AWVariant=Passthrough  PCopyVariant=Disabled  TRVariant=Disabled  FdbkBlocksVariant=Forward  IdealPFdbkVariant=Disabled  SatFdbkVariant=Disabled  DerivativeFilterVariant=Disabled  NVariant=Disabled  NCopyVariant=Disabled_SignalSpec  FilterICVariant=Disabled  IntegratorICVariant=InternalICs  ExternalResetVariant=Disabled  TRSumVariant=Passthrough  SumFdbkVariant=Disabled  SumVariant=Sum_PI
  Valve : Outport
  wires:
  T_err/1 -> PID Controller/1
  PID Controller/1 -> Valve/1

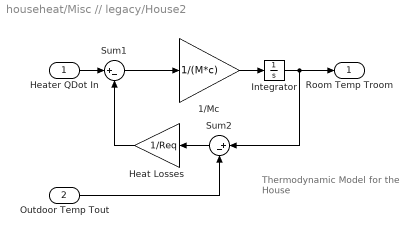
== system househeat/Misc // legacy/House2 ==
  note: Thermodynamic Model
      | for the House
  Heater QDot In : Inport
  Outdoor Temp Tout : Inport  Port=2
  1/Mc : Gain  Gain=1/(M*c)  SaturateOnIntegerOverflow=on  OutDataTypeStr=Inherit: Same as input  ParamDataTypeStr=Inherit: Same as input
  Heat Losses : Gain  Gain=1/Req  SaturateOnIntegerOverflow=on  OutDataTypeStr=Inherit: Same as input  ParamDataTypeStr=Inherit: Same as input
  Integrator : Integrator  InitialCondition=TinIC
  Sum1 : Sum  Inputs=|+-  SaturateOnIntegerOverflow=on  InputSameDT=on  OutDataTypeStr=Inherit: Same as first input
  Sum2 : Sum  Inputs=|+-  SaturateOnIntegerOverflow=on  InputSameDT=on  OutDataTypeStr=Inherit: Same as first input
  Room Temp Troom : Outport  InitialOutput=0
  wires:
  Outdoor Temp Tout/1 -> Sum2/2
  Heater QDot In/1 -> Sum1/1
  Sum1/1 -> 1/Mc/1
  Sum2/1 -> Heat Losses/1
  Heat Losses/1 -> Sum1/2
  1/Mc/1 -> Integrator/1
  Integrator/1 -> Sum2/1, Room Temp Troom/1

== system househeat/Misc // legacy/Thermostat ==
  note: Thermostat Subsystem
  Terr : Inport
  Relay1 : Relay  OnSwitchValue=1  OffSwitchValue=-1
  Blower switch : Outport  InitialOutput=0
  wires:
  Terr/1 -> Relay1/1
  Relay1/1 -> Blower switch/1

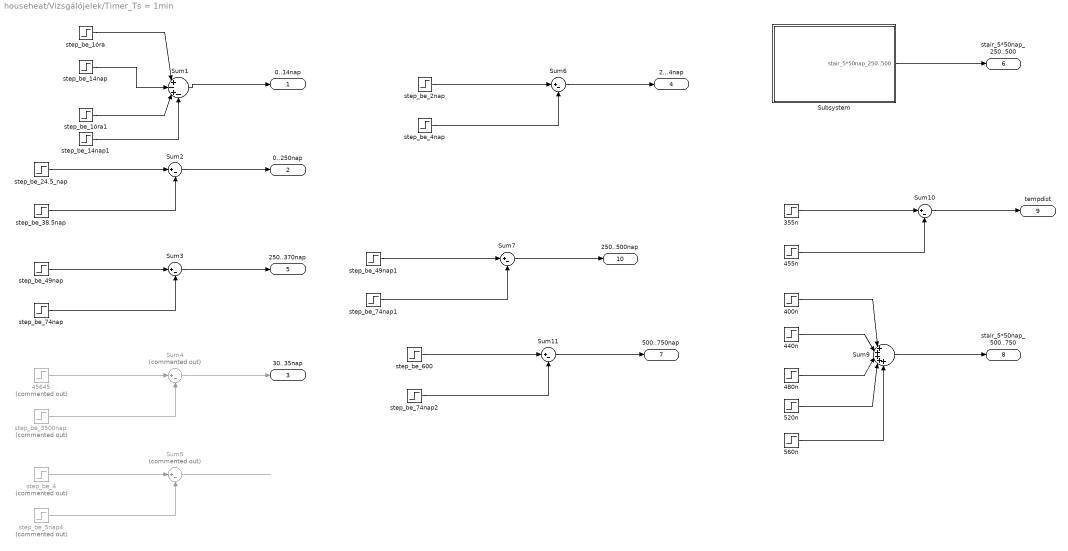
== system househeat/Vizsgálójelek/Timer_Ts = 1min ==
  355n : Step  Time=3600*24*10*45  After=15  SampleTime=T_s
  400n : Step  Time=3600*24*10*50  After=0.1  SampleTime=T_s
  440n : Step  Time=3600*24*10*54  After=0.1  SampleTime=T_s
  455n : Step  Time=3600*24*10*50  After=20  SampleTime=T_s
  45645 : Step  Commented=on  Time=3600*24*30  SampleTime=0
  480n : Step  Time=3600*24*10*58  After=0.1  SampleTime=T_s
  520n : Step  Time=3600*24*10*62  After=0.3  SampleTime=T_s
  560n : Step  Time=3600*24*10*66  After=0.4  SampleTime=T_s
  Subsystem : Subsystem
  Sum1 : Sum  Inputs=|+-+-  SaturateOnIntegerOverflow=on  InputSameDT=on  OutDataTypeStr=Inherit: Same as first input
  Sum{2..3,6..7,10..11} (6 alike) : Sum  Inputs=|+-  SaturateOnIntegerOverflow=on  InputSameDT=on  OutDataTypeStr=Inherit: Same as first input
  Sum4 : Sum  Commented=on  Inputs=|+-  SaturateOnIntegerOverflow=on  InputSameDT=on  OutDataTypeStr=Inherit: Same as first input
  Sum5 : Sum  Commented=on  Inputs=|+-  SaturateOnIntegerOverflow=on  InputSameDT=on  OutDataTypeStr=Inherit: Same as first input
  Sum9 : Sum  Inputs=|+++++  SaturateOnIntegerOverflow=on  InputSameDT=on  OutDataTypeStr=Inherit: Same as first input
  step_be_14nap : Step  Time=timeUnit_1week*7*T_s  SampleTime=T_s
  step_be_14nap1 : Step  Time=timeUnit_1week*20*T_s  SampleTime=T_s
  step_be_1óra : Step  Time=0  SampleTime=T_s
  step_be_1óra1 : Step  Time=timeUnit_1week*17*T_s  SampleTime=T_s
  step_be_24.5_nap : Step  Time=0  SampleTime=T_s
  step_be_2nap : Step  Time=3600*24*2  SampleTime=0
  step_be_3500nap : Step  Commented=on  Time=3600*24*35  SampleTime=0
  step_be_38.5nap : Step  Time=3600*24*10*25  SampleTime=T_s
  step_be_4 : Step  Commented=on  Time=0  SampleTime=0
  step_be_49nap : Step  Time=3600*24*10*25  SampleTime=T_s
  step_be_49nap1 : Step  Time=3600*24*10*25  SampleTime=T_s
  step_be_4nap : Step  Time=3600*24*4  SampleTime=0
  step_be_5nap4 : Step  Commented=on  Time=3600*24*5  SampleTime=0
  step_be_600 : Step  Time=3600*24*10*50  SampleTime=T_s
  step_be_74nap : Step  Time=3600*24*10*45  SampleTime=T_s
  step_be_74nap1 : Step  Time=3600*24*10*50  SampleTime=T_s
  step_be_74nap2 : Step  Time=3600*24*10*70  SampleTime=T_s
  0..14nap : Outport
  0..250nap : Outport  Port=2
  30..35nap : Outport  Port=3
  2...4nap : Outport  Port=4
  250..370nap : Outport  Port=5
  stair_5*50nap_250..500 : Outport  Port=6
  500..750nap : Outport  Port=7
  stair_5*50nap_500..750 : Outport  Port=8
  tempdist : Outport  Port=9
  250..500nap : Outport  Port=10
  wires:
  Sum1/1 -> 0..14nap/1
  step_be_14nap/1 -> Sum1/2
  step_be_1óra/1 -> Sum1/1
  Sum2/1 -> 0..250nap/1
  step_be_38.5nap/1 -> Sum2/2
  step_be_24.5_nap/1 -> Sum2/1
  Sum3/1 -> 250..370nap/1
  step_be_74nap/1 -> Sum3/2
  step_be_49nap/1 -> Sum3/1
  Sum4/1 -> 30..35nap/1
  step_be_3500nap/1 -> Sum4/2
  45645/1 -> Sum4/1
  Sum5/1 -> ?
  step_be_5nap4/1 -> Sum5/2
  step_be_4/1 -> Sum5/1
  Sum6/1 -> 2...4nap/1
  step_be_4nap/1 -> Sum6/2
  step_be_2nap/1 -> Sum6/1
  step_be_14nap1/1 -> Sum1/4
  step_be_1óra1/1 -> Sum1/3
  Sum7/1 -> 250..500nap/1
  step_be_74nap1/1 -> Sum7/2
  step_be_49nap1/1 -> Sum7/1
  Sum9/1 -> stair_5*50nap_500..750/1
  440n/1 -> Sum9/2
  400n/1 -> Sum9/1
  520n/1 -> Sum9/4
  480n/1 -> Sum9/3
  560n/1 -> Sum9/5
  Sum10/1 -> tempdist/1
  455n/1 -> Sum10/2
  355n/1 -> Sum10/1
  Sum11/1 -> 500..750nap/1
  step_be_74nap2/1 -> Sum11/2
  step_be_600/1 -> Sum11/1
  Subsystem/1(stair_5*50nap_250..500) -> stair_5*50nap_250..500/1

== system househeat/Fűtőtestek/Padlofutes_thermal/Hőmérséklet-különbség ==
  Delay : Delay  DelayLength=1  InitialCondition=0
  Hőmérő 1 : Subsystem
  Hőmérő 2 : Subsystem
  Subtract : Sum  Inputs=+-
  in : PMIOPort  Side=Left
  in2 : PMIOPort  Port=2  Side=Left
  o1 : Outport
  o2 : Outport  Port=2
  wires:
  Subtract/1 -> Delay/1
  Hőmérő 2/1(T) -> o1/1, Subtract/1
  Hőmérő 1/1(T) -> Subtract/2
  Delay/1 -> o2/1
  connections:
  Hőmérő 1/LConn1 -- in/RConn1
  Hőmérő 2/LConn1 -- in2/RConn1

== system househeat/Fűtőtestek/Subsystem/Hőmérő 1 ==
  PS2S : nesl_utility/PS-Simulink Converter  PhysicalDomain=network_engine_domain  SubClassName=ps_output  LeftPortType=input  RightPortType=output  PseudoPeriodic=off  Frequencies=[]  Unit=degC  AffineConversion=on
  TRef : fl_lib/Thermal/Thermal Elements/Thermal Reference
  Temperature Sensor : fl_lib/Thermal/Thermal Sensors/Temperature Sensor
  Pr : PMIOPort  Side=Left
  T : Outport
  wires:
  PS2S/1 -> T/1
  connections:
  Temperature Sensor/RConn1 -- TRef/LConn1
  PS2S/LConn1 -- Temperature Sensor/RConn2
  Pr/RConn1 -- Temperature Sensor/LConn1

== system househeat/Fűtőtestek/Subsystem/Hőmérő 2 ==
  PS2S : nesl_utility/PS-Simulink Converter  PhysicalDomain=network_engine_domain  SubClassName=ps_output  LeftPortType=input  RightPortType=output  PseudoPeriodic=off  Frequencies=[]  Unit=degC  AffineConversion=on
  TRef : fl_lib/Thermal/Thermal Elements/Thermal Reference
  Temperature Sensor : fl_lib/Thermal/Thermal Sensors/Temperature Sensor
  Pr : PMIOPort  Side=Left
  T : Outport
  wires:
  PS2S/1 -> T/1
  connections:
  Temperature Sensor/RConn1 -- TRef/LConn1
  PS2S/LConn1 -- Temperature Sensor/RConn2
  Pr/RConn1 -- Temperature Sensor/LConn1

== system househeat/Helyiség/House Simscape/Hőmérő 1 ==
  PS2S : nesl_utility/PS-Simulink Converter  PhysicalDomain=network_engine_domain  SubClassName=ps_output  LeftPortType=input  RightPortType=output  PseudoPeriodic=off  Frequencies=[]  Unit=degC  AffineConversion=on
  TRef : fl_lib/Thermal/Thermal Elements/Thermal Reference
  Temperature Sensor : fl_lib/Thermal/Thermal Sensors/Temperature Sensor
  Pr : PMIOPort  Side=Left
  T : Outport
  wires:
  PS2S/1 -> T/1
  connections:
  Temperature Sensor/RConn1 -- TRef/LConn1
  PS2S/LConn1 -- Temperature Sensor/RConn2
  Pr/RConn1 -- Temperature Sensor/LConn1

== system househeat/Helyiség/House Simscape/Hőmérő 2 ==
  PS2S : nesl_utility/PS-Simulink Converter  PhysicalDomain=network_engine_domain  SubClassName=ps_output  LeftPortType=input  RightPortType=output  PseudoPeriodic=off  Frequencies=[]  Unit=K  AffineConversion=on
  TRef : fl_lib/Thermal/Thermal Elements/Thermal Reference
  Temperature Sensor : fl_lib/Thermal/Thermal Sensors/Temperature Sensor
  Pr : PMIOPort  Side=Left
  T_i [K] : Outport
  wires:
  PS2S/1 -> T_i [K]/1
  connections:
  Temperature Sensor/RConn1 -- TRef/LConn1
  PS2S/LConn1 -- Temperature Sensor/RConn2
  Pr/RConn1 -- Temperature Sensor/LConn1

== system househeat/Vizsgálójelek/Timer_Ts = 1min/Subsystem ==
  250n : Step  Time=3600*24*10*25  After=0.1  SampleTime=T_s
  280n : Step  Time=3600*24*10*29  After=0.1  SampleTime=T_s
  310n : Step  Time=3600*24*10*33  After=0.2  SampleTime=T_s
  340n : Step  Time=3600*24*10*37  After=0.2  SampleTime=T_s
  370n : Step  Time=3600*24*10*41  After=0.4  SampleTime=T_s
  Sum8 : Sum  Inputs=|+++++  SaturateOnIntegerOverflow=on  InputSameDT=on  OutDataTypeStr=Inherit: Same as first input
  stair_5*50nap_250..500 : Outport
  wires:
  370n/1 -> Sum8/5
  280n/1 -> Sum8/2
  340n/1 -> Sum8/4
  310n/1 -> Sum8/3
  250n/1 -> Sum8/1
  Sum8/1 -> stair_5*50nap_250..500/1

== system househeat/Fűtőtestek/Padlofutes_thermal/Hőmérséklet-különbség/Hőmérő 1 ==
  PS2S : nesl_utility/PS-Simulink Converter  PhysicalDomain=network_engine_domain  SubClassName=ps_output  LeftPortType=input  RightPortType=output  PseudoPeriodic=off  Frequencies=[]  Unit=degC  AffineConversion=on
  TRef : fl_lib/Thermal/Thermal Elements/Thermal Reference
  Temperature Sensor : fl_lib/Thermal/Thermal Sensors/Temperature Sensor
  Pr : PMIOPort  Side=Left
  T : Outport
  wires:
  PS2S/1 -> T/1
  connections:
  Temperature Sensor/RConn1 -- TRef/LConn1
  PS2S/LConn1 -- Temperature Sensor/RConn2
  Pr/RConn1 -- Temperature Sensor/LConn1

== system househeat/Fűtőtestek/Padlofutes_thermal/Hőmérséklet-különbség/Hőmérő 2 ==
  PS2S : nesl_utility/PS-Simulink Converter  PhysicalDomain=network_engine_domain  SubClassName=ps_output  LeftPortType=input  RightPortType=output  PseudoPeriodic=off  Frequencies=[]  Unit=degC  AffineConversion=on
  TRef : fl_lib/Thermal/Thermal Elements/Thermal Reference
  Temperature Sensor : fl_lib/Thermal/Thermal Sensors/Temperature Sensor
  Pr : PMIOPort  Side=Left
  T : Outport
  wires:
  PS2S/1 -> T/1
  connections:
  Temperature Sensor/RConn1 -- TRef/LConn1
  PS2S/LConn1 -- Temperature Sensor/RConn2
  Pr/RConn1 -- Temperature Sensor/LConn1

== matlab function househeat/Reference Previewer2/MATLAB Function ==
  settings: updateMethod=DISCRETE  sampleTime=ts
  data: data parameter double; seq output double; steps parameter double; t input double; first output double; next_t output double
function [seq,first,next_t] = fcn(data,steps,t)
%#codegen
[seq,first,next_t] = mpcblock_preview('ref',data,steps,t);

== matlab function househeat/Disturbance Preview/MATLAB Function ==
  settings: updateMethod=DISCRETE  sampleTime=ts
  data: data parameter double; seq output double; steps parameter double; t input double; first output double; next_t output double
function [seq,first,next_t] = fcn(data,steps,t)
%#codegen
[seq,first,next_t] = mpcblock_preview('ref',data,steps,t);
